simulink subsystem "SPWM_modulator"  (R2022b)
settings: Solver=VariableStepAuto  StartTime=0.0  StopTime=10.0  RelTol=1e-3
libraries: spsTriangleGeneratorLib x1
settings Model: Creator=jack  LastModifiedBy=jack

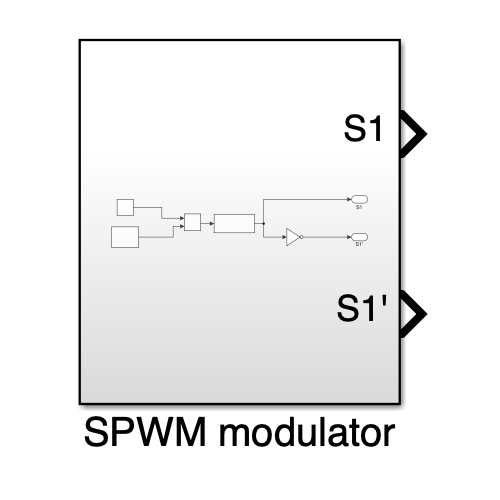
[thumbnail: Simulink's stored preview of the top-level diagram]
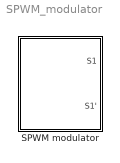
== system SPWM_modulator ==
  SPWM modulator : Subsystem

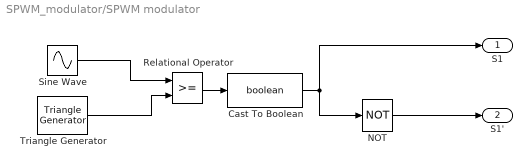
== system SPWM_modulator/SPWM modulator ==
  Cast To Boolean : DataTypeConversion  OutDataTypeStr=boolean  SaturateOnIntegerOverflow=off  RndMeth=Floor
  NOT : Logic  Operator=NOT  IconShape=distinctive  AllPortsSameDT=off  OutDataTypeStr=boolean
  Relational Operator : RelationalOperator  OutDataTypeStr=boolean  RndMeth=Simplest  InputSameDT=off
  Sine Wave : Sin  Frequency=2*pi*50  SampleTime=0
  Triangle Generator : spsTriangleGeneratorLib/Triangle Generator  Freq=2e3  Phase=90  Ts=0
  S1 : Outport
  S1' : Outport  Port=2
  wires:
  Relational Operator/1 -> Cast To Boolean/1
  NOT/1 -> S1'/1
  Triangle Generator/1 -> Relational Operator/2
  Cast To Boolean/1 -> S1/1, NOT/1
  Sine Wave/1 -> Relational Operator/1
